simulink model "IP_Core_SS_Switch_and_PWM"  (R2021a)
settings: Solver=VariableStepAuto  StartTime=0.0  StopTime=0.05  RelTol=1e-3
undefined symbols (not defined in the file): f_FPGA_clk, T_FPGA_clk
libraries: hdlsllib x2
(part 2 of 2)

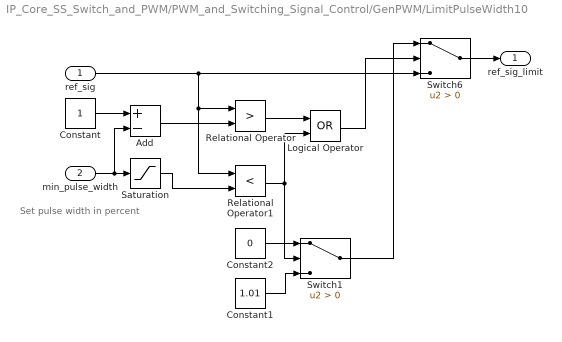
== system IP_Core_SS_Switch_and_PWM/PWM_and_Switching_Signal_Control/GenPWM/LimitPulseWidth10 ==
  note: Set pulse width in percent
  ref_sig : Inport
  min_pulse_width : Inport  Port=2
  Add : Sum  Inputs=+-  OutDataTypeStr=Inherit: Same as first input
  Constant : Constant  OutDataTypeStr=fixdt(1,18,16)  SampleTime=T_FPGA_clk
  Constant1 : Constant  Value=1.01  OutDataTypeStr=fixdt(1,18,16)  SampleTime=T_FPGA_clk
  Constant2 : Constant  Value=0  OutDataTypeStr=fixdt(1,18,16)  SampleTime=T_FPGA_clk
  Logical Operator : Logic  Operator=OR  AllPortsSameDT=off  OutDataTypeStr=boolean
  Relational Operator : RelationalOperator  Operator=>  OutDataTypeStr=boolean  RndMeth=Nearest
  Relational Operator1 : RelationalOperator  Operator=<  OutDataTypeStr=boolean  RndMeth=Nearest
  Saturation : Saturate  UpperLimit=1  LowerLimit=0  OutDataTypeStr=fixdt(1,18,16)
  Switch1 : Switch  Criteria=u2 > Threshold
  Switch6 : Switch  Criteria=u2 > Threshold
  ref_sig_limit : Outport  VectorParamsAs1DForOutWhenUnconnected=off
  wires:
  Constant/1 -> Add/1
  min_pulse_width/1 -> Add/2, Saturation/1
  Add/1 -> Relational Operator/2
  ref_sig/1 -> Switch6/3, Relational Operator/1, Relational Operator1/1
  Relational Operator/1 -> Logical Operator/1
  Relational Operator1/1 -> Logical Operator/2, Switch1/2
  Logical Operator/1 -> Switch6/2
  Constant1/1 -> Switch1/3
  Switch1/1 -> Switch6/1
  Constant2/1 -> Switch1/1
  Switch6/1 -> ref_sig_limit/1
  Saturation/1 -> Relational Operator1/2

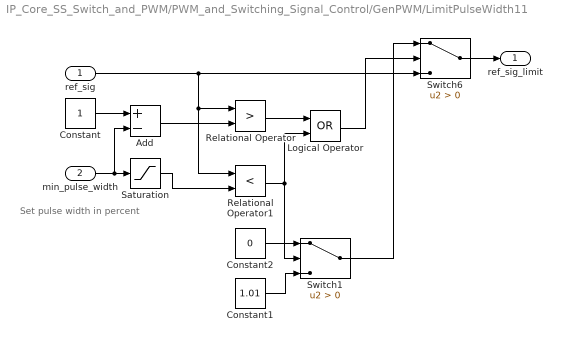
== system IP_Core_SS_Switch_and_PWM/PWM_and_Switching_Signal_Control/GenPWM/LimitPulseWidth11 ==
  note: Set pulse width in percent
  ref_sig : Inport
  min_pulse_width : Inport  Port=2
  Add : Sum  Inputs=+-  OutDataTypeStr=Inherit: Same as first input
  Constant : Constant  OutDataTypeStr=fixdt(1,18,16)  SampleTime=T_FPGA_clk
  Constant1 : Constant  Value=1.01  OutDataTypeStr=fixdt(1,18,16)  SampleTime=T_FPGA_clk
  Constant2 : Constant  Value=0  OutDataTypeStr=fixdt(1,18,16)  SampleTime=T_FPGA_clk
  Logical Operator : Logic  Operator=OR  AllPortsSameDT=off  OutDataTypeStr=boolean
  Relational Operator : RelationalOperator  Operator=>  OutDataTypeStr=boolean  RndMeth=Nearest
  Relational Operator1 : RelationalOperator  Operator=<  OutDataTypeStr=boolean  RndMeth=Nearest
  Saturation : Saturate  UpperLimit=1  LowerLimit=0  OutDataTypeStr=fixdt(1,18,16)
  Switch1 : Switch  Criteria=u2 > Threshold
  Switch6 : Switch  Criteria=u2 > Threshold
  ref_sig_limit : Outport  VectorParamsAs1DForOutWhenUnconnected=off
  wires:
  Constant/1 -> Add/1
  min_pulse_width/1 -> Add/2, Saturation/1
  Add/1 -> Relational Operator/2
  ref_sig/1 -> Switch6/3, Relational Operator/1, Relational Operator1/1
  Relational Operator/1 -> Logical Operator/1
  Relational Operator1/1 -> Logical Operator/2, Switch1/2
  Logical Operator/1 -> Switch6/2
  Constant1/1 -> Switch1/3
  Switch1/1 -> Switch6/1
  Constant2/1 -> Switch1/1
  Switch6/1 -> ref_sig_limit/1
  Saturation/1 -> Relational Operator1/2

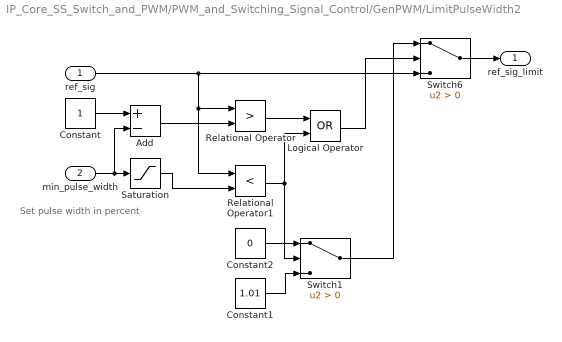
== system IP_Core_SS_Switch_and_PWM/PWM_and_Switching_Signal_Control/GenPWM/LimitPulseWidth2 ==
  note: Set pulse width in percent
  ref_sig : Inport
  min_pulse_width : Inport  Port=2
  Add : Sum  Inputs=+-  OutDataTypeStr=Inherit: Same as first input
  Constant : Constant  OutDataTypeStr=fixdt(1,18,16)  SampleTime=T_FPGA_clk
  Constant1 : Constant  Value=1.01  OutDataTypeStr=fixdt(1,18,16)  SampleTime=T_FPGA_clk
  Constant2 : Constant  Value=0  OutDataTypeStr=fixdt(1,18,16)  SampleTime=T_FPGA_clk
  Logical Operator : Logic  Operator=OR  AllPortsSameDT=off  OutDataTypeStr=boolean
  Relational Operator : RelationalOperator  Operator=>  OutDataTypeStr=boolean  RndMeth=Nearest
  Relational Operator1 : RelationalOperator  Operator=<  OutDataTypeStr=boolean  RndMeth=Nearest
  Saturation : Saturate  UpperLimit=1  LowerLimit=0  OutDataTypeStr=fixdt(1,18,16)
  Switch1 : Switch  Criteria=u2 > Threshold
  Switch6 : Switch  Criteria=u2 > Threshold
  ref_sig_limit : Outport  VectorParamsAs1DForOutWhenUnconnected=off
  wires:
  Constant/1 -> Add/1
  min_pulse_width/1 -> Add/2, Saturation/1
  Add/1 -> Relational Operator/2
  ref_sig/1 -> Switch6/3, Relational Operator/1, Relational Operator1/1
  Relational Operator/1 -> Logical Operator/1
  Relational Operator1/1 -> Logical Operator/2, Switch1/2
  Logical Operator/1 -> Switch6/2
  Constant1/1 -> Switch1/3
  Switch1/1 -> Switch6/1
  Constant2/1 -> Switch1/1
  Switch6/1 -> ref_sig_limit/1
  Saturation/1 -> Relational Operator1/2

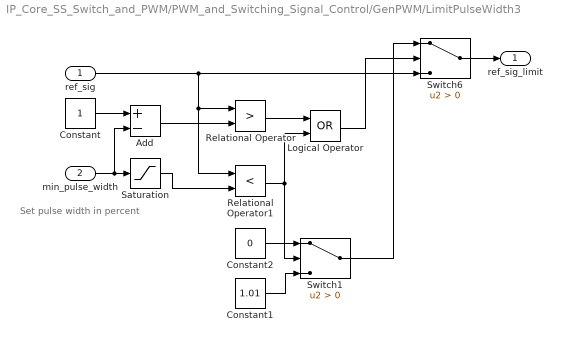
== system IP_Core_SS_Switch_and_PWM/PWM_and_Switching_Signal_Control/GenPWM/LimitPulseWidth3 ==
  note: Set pulse width in percent
  ref_sig : Inport
  min_pulse_width : Inport  Port=2
  Add : Sum  Inputs=+-  OutDataTypeStr=Inherit: Same as first input
  Constant : Constant  OutDataTypeStr=fixdt(1,18,16)  SampleTime=T_FPGA_clk
  Constant1 : Constant  Value=1.01  OutDataTypeStr=fixdt(1,18,16)  SampleTime=T_FPGA_clk
  Constant2 : Constant  Value=0  OutDataTypeStr=fixdt(1,18,16)  SampleTime=T_FPGA_clk
  Logical Operator : Logic  Operator=OR  AllPortsSameDT=off  OutDataTypeStr=boolean
  Relational Operator : RelationalOperator  Operator=>  OutDataTypeStr=boolean  RndMeth=Nearest
  Relational Operator1 : RelationalOperator  Operator=<  OutDataTypeStr=boolean  RndMeth=Nearest
  Saturation : Saturate  UpperLimit=1  LowerLimit=0  OutDataTypeStr=fixdt(1,18,16)
  Switch1 : Switch  Criteria=u2 > Threshold
  Switch6 : Switch  Criteria=u2 > Threshold
  ref_sig_limit : Outport  VectorParamsAs1DForOutWhenUnconnected=off
  wires:
  Constant/1 -> Add/1
  min_pulse_width/1 -> Add/2, Saturation/1
  Add/1 -> Relational Operator/2
  ref_sig/1 -> Switch6/3, Relational Operator/1, Relational Operator1/1
  Relational Operator/1 -> Logical Operator/1
  Relational Operator1/1 -> Logical Operator/2, Switch1/2
  Logical Operator/1 -> Switch6/2
  Constant1/1 -> Switch1/3
  Switch1/1 -> Switch6/1
  Constant2/1 -> Switch1/1
  Switch6/1 -> ref_sig_limit/1
  Saturation/1 -> Relational Operator1/2

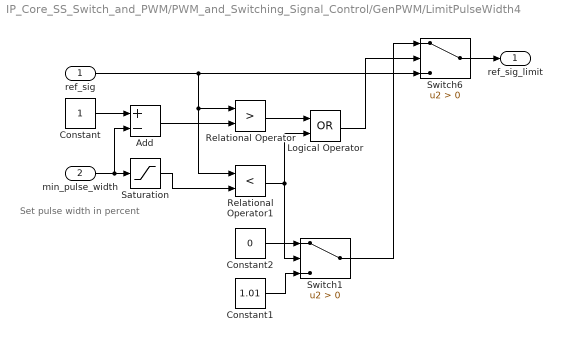
== system IP_Core_SS_Switch_and_PWM/PWM_and_Switching_Signal_Control/GenPWM/LimitPulseWidth4 ==
  note: Set pulse width in percent
  ref_sig : Inport
  min_pulse_width : Inport  Port=2
  Add : Sum  Inputs=+-  OutDataTypeStr=Inherit: Same as first input
  Constant : Constant  OutDataTypeStr=fixdt(1,18,16)  SampleTime=T_FPGA_clk
  Constant1 : Constant  Value=1.01  OutDataTypeStr=fixdt(1,18,16)  SampleTime=T_FPGA_clk
  Constant2 : Constant  Value=0  OutDataTypeStr=fixdt(1,18,16)  SampleTime=T_FPGA_clk
  Logical Operator : Logic  Operator=OR  AllPortsSameDT=off  OutDataTypeStr=boolean
  Relational Operator : RelationalOperator  Operator=>  OutDataTypeStr=boolean  RndMeth=Nearest
  Relational Operator1 : RelationalOperator  Operator=<  OutDataTypeStr=boolean  RndMeth=Nearest
  Saturation : Saturate  UpperLimit=1  LowerLimit=0  OutDataTypeStr=fixdt(1,18,16)
  Switch1 : Switch  Criteria=u2 > Threshold
  Switch6 : Switch  Criteria=u2 > Threshold
  ref_sig_limit : Outport  VectorParamsAs1DForOutWhenUnconnected=off
  wires:
  Constant/1 -> Add/1
  min_pulse_width/1 -> Add/2, Saturation/1
  Add/1 -> Relational Operator/2
  ref_sig/1 -> Switch6/3, Relational Operator/1, Relational Operator1/1
  Relational Operator/1 -> Logical Operator/1
  Relational Operator1/1 -> Logical Operator/2, Switch1/2
  Logical Operator/1 -> Switch6/2
  Constant1/1 -> Switch1/3
  Switch1/1 -> Switch6/1
  Constant2/1 -> Switch1/1
  Switch6/1 -> ref_sig_limit/1
  Saturation/1 -> Relational Operator1/2

== system IP_Core_SS_Switch_and_PWM/PWM_and_Switching_Signal_Control/GenPWM/LimitPulseWidth5 ==
  note: Set pulse width in percent
  ref_sig : Inport
  min_pulse_width : Inport  Port=2
  Add : Sum  Inputs=+-  OutDataTypeStr=Inherit: Same as first input
  Constant : Constant  OutDataTypeStr=fixdt(1,18,16)  SampleTime=T_FPGA_clk
  Constant1 : Constant  Value=1.01  OutDataTypeStr=fixdt(1,18,16)  SampleTime=T_FPGA_clk
  Constant2 : Constant  Value=0  OutDataTypeStr=fixdt(1,18,16)  SampleTime=T_FPGA_clk
  Logical Operator : Logic  Operator=OR  AllPortsSameDT=off  OutDataTypeStr=boolean
  Relational Operator : RelationalOperator  Operator=>  OutDataTypeStr=boolean  RndMeth=Nearest
  Relational Operator1 : RelationalOperator  Operator=<  OutDataTypeStr=boolean  RndMeth=Nearest
  Saturation : Saturate  UpperLimit=1  LowerLimit=0  OutDataTypeStr=fixdt(1,18,16)
  Switch1 : Switch  Criteria=u2 > Threshold
  Switch6 : Switch  Criteria=u2 > Threshold
  ref_sig_limit : Outport  VectorParamsAs1DForOutWhenUnconnected=off
  wires:
  Constant/1 -> Add/1
  min_pulse_width/1 -> Add/2, Saturation/1
  Add/1 -> Relational Operator/2
  ref_sig/1 -> Switch6/3, Relational Operator/1, Relational Operator1/1
  Relational Operator/1 -> Logical Operator/1
  Relational Operator1/1 -> Logical Operator/2, Switch1/2
  Logical Operator/1 -> Switch6/2
  Constant1/1 -> Switch1/3
  Switch1/1 -> Switch6/1
  Constant2/1 -> Switch1/1
  Switch6/1 -> ref_sig_limit/1
  Saturation/1 -> Relational Operator1/2

== system IP_Core_SS_Switch_and_PWM/PWM_and_Switching_Signal_Control/GenPWM/LimitPulseWidth6 ==
  note: Set pulse width in percent
  ref_sig : Inport
  min_pulse_width : Inport  Port=2
  Add : Sum  Inputs=+-  OutDataTypeStr=Inherit: Same as first input
  Constant : Constant  OutDataTypeStr=fixdt(1,18,16)  SampleTime=T_FPGA_clk
  Constant1 : Constant  Value=1.01  OutDataTypeStr=fixdt(1,18,16)  SampleTime=T_FPGA_clk
  Constant2 : Constant  Value=0  OutDataTypeStr=fixdt(1,18,16)  SampleTime=T_FPGA_clk
  Logical Operator : Logic  Operator=OR  AllPortsSameDT=off  OutDataTypeStr=boolean
  Relational Operator : RelationalOperator  Operator=>  OutDataTypeStr=boolean  RndMeth=Nearest
  Relational Operator1 : RelationalOperator  Operator=<  OutDataTypeStr=boolean  RndMeth=Nearest
  Saturation : Saturate  UpperLimit=1  LowerLimit=0  OutDataTypeStr=fixdt(1,18,16)
  Switch1 : Switch  Criteria=u2 > Threshold
  Switch6 : Switch  Criteria=u2 > Threshold
  ref_sig_limit : Outport  VectorParamsAs1DForOutWhenUnconnected=off
  wires:
  Constant/1 -> Add/1
  min_pulse_width/1 -> Add/2, Saturation/1
  Add/1 -> Relational Operator/2
  ref_sig/1 -> Switch6/3, Relational Operator/1, Relational Operator1/1
  Relational Operator/1 -> Logical Operator/1
  Relational Operator1/1 -> Logical Operator/2, Switch1/2
  Logical Operator/1 -> Switch6/2
  Constant1/1 -> Switch1/3
  Switch1/1 -> Switch6/1
  Constant2/1 -> Switch1/1
  Switch6/1 -> ref_sig_limit/1
  Saturation/1 -> Relational Operator1/2

== system IP_Core_SS_Switch_and_PWM/PWM_and_Switching_Signal_Control/GenPWM/LimitPulseWidth7 ==
  note: Set pulse width in percent
  ref_sig : Inport
  min_pulse_width : Inport  Port=2
  Add : Sum  Inputs=+-  OutDataTypeStr=Inherit: Same as first input
  Constant : Constant  OutDataTypeStr=fixdt(1,18,16)  SampleTime=T_FPGA_clk
  Constant1 : Constant  Value=1.01  OutDataTypeStr=fixdt(1,18,16)  SampleTime=T_FPGA_clk
  Constant2 : Constant  Value=0  OutDataTypeStr=fixdt(1,18,16)  SampleTime=T_FPGA_clk
  Logical Operator : Logic  Operator=OR  AllPortsSameDT=off  OutDataTypeStr=boolean
  Relational Operator : RelationalOperator  Operator=>  OutDataTypeStr=boolean  RndMeth=Nearest
  Relational Operator1 : RelationalOperator  Operator=<  OutDataTypeStr=boolean  RndMeth=Nearest
  Saturation : Saturate  UpperLimit=1  LowerLimit=0  OutDataTypeStr=fixdt(1,18,16)
  Switch1 : Switch  Criteria=u2 > Threshold
  Switch6 : Switch  Criteria=u2 > Threshold
  ref_sig_limit : Outport  VectorParamsAs1DForOutWhenUnconnected=off
  wires:
  Constant/1 -> Add/1
  min_pulse_width/1 -> Add/2, Saturation/1
  Add/1 -> Relational Operator/2
  ref_sig/1 -> Switch6/3, Relational Operator/1, Relational Operator1/1
  Relational Operator/1 -> Logical Operator/1
  Relational Operator1/1 -> Logical Operator/2, Switch1/2
  Logical Operator/1 -> Switch6/2
  Constant1/1 -> Switch1/3
  Switch1/1 -> Switch6/1
  Constant2/1 -> Switch1/1
  Switch6/1 -> ref_sig_limit/1
  Saturation/1 -> Relational Operator1/2

== system IP_Core_SS_Switch_and_PWM/PWM_and_Switching_Signal_Control/GenPWM/LimitPulseWidth8 ==
  note: Set pulse width in percent
  ref_sig : Inport
  min_pulse_width : Inport  Port=2
  Add : Sum  Inputs=+-  OutDataTypeStr=Inherit: Same as first input
  Constant : Constant  OutDataTypeStr=fixdt(1,18,16)  SampleTime=T_FPGA_clk
  Constant1 : Constant  Value=1.01  OutDataTypeStr=fixdt(1,18,16)  SampleTime=T_FPGA_clk
  Constant2 : Constant  Value=0  OutDataTypeStr=fixdt(1,18,16)  SampleTime=T_FPGA_clk
  Logical Operator : Logic  Operator=OR  AllPortsSameDT=off  OutDataTypeStr=boolean
  Relational Operator : RelationalOperator  Operator=>  OutDataTypeStr=boolean  RndMeth=Nearest
  Relational Operator1 : RelationalOperator  Operator=<  OutDataTypeStr=boolean  RndMeth=Nearest
  Saturation : Saturate  UpperLimit=1  LowerLimit=0  OutDataTypeStr=fixdt(1,18,16)
  Switch1 : Switch  Criteria=u2 > Threshold
  Switch6 : Switch  Criteria=u2 > Threshold
  ref_sig_limit : Outport  VectorParamsAs1DForOutWhenUnconnected=off
  wires:
  Constant/1 -> Add/1
  min_pulse_width/1 -> Add/2, Saturation/1
  Add/1 -> Relational Operator/2
  ref_sig/1 -> Switch6/3, Relational Operator/1, Relational Operator1/1
  Relational Operator/1 -> Logical Operator/1
  Relational Operator1/1 -> Logical Operator/2, Switch1/2
  Logical Operator/1 -> Switch6/2
  Constant1/1 -> Switch1/3
  Switch1/1 -> Switch6/1
  Constant2/1 -> Switch1/1
  Switch6/1 -> ref_sig_limit/1
  Saturation/1 -> Relational Operator1/2

== system IP_Core_SS_Switch_and_PWM/PWM_and_Switching_Signal_Control/GenPWM/LimitPulseWidth9 ==
  note: Set pulse width in percent
  ref_sig : Inport
  min_pulse_width : Inport  Port=2
  Add : Sum  Inputs=+-  OutDataTypeStr=Inherit: Same as first input
  Constant : Constant  OutDataTypeStr=fixdt(1,18,16)  SampleTime=T_FPGA_clk
  Constant1 : Constant  Value=1.01  OutDataTypeStr=fixdt(1,18,16)  SampleTime=T_FPGA_clk
  Constant2 : Constant  Value=0  OutDataTypeStr=fixdt(1,18,16)  SampleTime=T_FPGA_clk
  Logical Operator : Logic  Operator=OR  AllPortsSameDT=off  OutDataTypeStr=boolean
  Relational Operator : RelationalOperator  Operator=>  OutDataTypeStr=boolean  RndMeth=Nearest
  Relational Operator1 : RelationalOperator  Operator=<  OutDataTypeStr=boolean  RndMeth=Nearest
  Saturation : Saturate  UpperLimit=1  LowerLimit=0  OutDataTypeStr=fixdt(1,18,16)
  Switch1 : Switch  Criteria=u2 > Threshold
  Switch6 : Switch  Criteria=u2 > Threshold
  ref_sig_limit : Outport  VectorParamsAs1DForOutWhenUnconnected=off
  wires:
  Constant/1 -> Add/1
  min_pulse_width/1 -> Add/2, Saturation/1
  Add/1 -> Relational Operator/2
  ref_sig/1 -> Switch6/3, Relational Operator/1, Relational Operator1/1
  Relational Operator/1 -> Logical Operator/1
  Relational Operator1/1 -> Logical Operator/2, Switch1/2
  Logical Operator/1 -> Switch6/2
  Constant1/1 -> Switch1/3
  Switch1/1 -> Switch6/1
  Constant2/1 -> Switch1/1
  Switch6/1 -> ref_sig_limit/1
  Saturation/1 -> Relational Operator1/2
